simulink model "ModeAdjust"  (R2018b)
settings: Solver=FixedStepDiscrete  StartTime=0.0  StopTime=inf  FixedStep=0.01  RelTol=1e-3
undefined symbols (not defined in the file or in its folder): IfKeSMSbSeatMovBkRclnEnable_Val, IfKeSMSbSeatMovFrwdBkwdEnable_Val, IfKeSMSbSeatMovFtrstEnable_Val, IfKeSMSbSeatMovHdrstFrwdBkwdEnable_Val, IfKeSMSbSeatMovHdUpwdDnwdEnable_Val, IfKeSMSbSeatMovLgrstEnable_Val, IfKeSMSbSeatMovLtwdRtwdEnable_Val, IfVeSMSeStNumConfig, KeSMSbArmscreenMovEnable_Val, KeSMSbSeatMovLgrstExpdEnable_Val, KeSMSuFirstRwStBackPosDelta_Val, KeSMSuFirstRwStBackPosTolr_Val, KeSMSuFirstRwStCushFrntPosDelta_Val, KeSMSuFirstRwStCushFrntPosTolr_Val, KeSMSuFirstRwStCushRePosDelta_Val, KeSMSuFirstRwStCushRePosTolr_Val, KeSMSuFirstRwStFootrestPosDelta_Val, KeSMSuFirstRwStFootrestPosTolr_Val, KeSMSuFirstRwStFwdBkwdPosDelta_Val, KeSMSuFirstRwStFwdBkwdPosTolr_Val, KeSMSuMdMotFinshdTm_Val, KeSMSuMdRetryTm1_Val, KeSMSuModeReqDurgTm_Val, KeSMSuSecRwStArmTochPosDelta_Val, KeSMSuSecRwStArmTochPosTolr_Val, KeSMSuSecRwStBackPosDelta_Val, KeSMSuSecRwStBackPosTolr_Val, KeSMSuSecRwStFtrstUpwdDnwdPosDelta_Val, KeSMSuSecRwStFtrstUpwdDnwdPosTolr_Val, KeSMSuSecRwStFwdBkwdPosDelta_Val, KeSMSuSecRwStFwdBkwdPosTolr_Val, KeSMSuSecRwStHeadrestFwdBkwdPosDelta_Val, KeSMSuSecRwStHeadrestFwdBkwdPosTolr_Val, KeSMSuSecRwStHeadrestUpwdDwnwdPosDelta_Val, KeSMSuSecRwStHeadrestUpwdDwnwdPosTolr_Val, KeSMSuSecRwStLegrestInOutPosDelta_Val, KeSMSuSecRwStLegrestInOutPosTolr_Val, KeSMSuSecRwStLegrestUpwdDwnwdPosDelta_Val, KeSMSuSecRwStLegrestUpwdDwnwdPosTolr_Val, KeSMSuSecRwStLwdRwdPosDelta_Val, KeSMSuSecRwStLwdRwdPosTolr_Val, KeSMSuSecRwStVIPFtrstRefAngle_Val, KeSMSuThirdRwStFwdBkwdPosDelta_Val, KeSMSuThirdRwStFwdBkwdPosTolr_Val, KeSMSuThrdRwCushFoldPosDelta_Val, KeSMSuThrdRwCushFoldPosTolr_Val, KeSMSuThrdRwStBackPosDelta_Val, KeSMSuThrdRwStBackPosTolr_Val, KeSMSw4SLegrstCloseMdSecRwLtStFtrstUpwdDnwdPos_Val, KeSMSw4SLegrstCloseMdSecRwLtStFtrstUpwdDnwdPosMax_Val, KeSMSw4SLegrstCloseMdSecRwLtStFtrstUpwdDnwdPosMin_Val, KeSMSw4SLegrstCloseMdSecRwLtStLgrstOtwdInwdPos_Val, KeSMSw4SLegrstCloseMdSecRwLtStLgrstOtwdInwdPosMax_Val, KeSMSw4SLegrstCloseMdSecRwLtStLgrstOtwdInwdPosMin_Val, KeSMSw4SLegrstCloseMdSecRwLtStLgrstUpwdDnwdPos_Val, KeSMSw4SLegrstCloseMdSecRwLtStLgrstUpwdDnwdPosMax_Val, KeSMSw4SLegrstCloseMdSecRwLtStLgrstUpwdDnwdPosMin_Val, KeSMSw4SLegrstCloseMdSecRwRtStFtrstUpwdDnwdPos_Val, KeSMSw4SLegrstCloseMdSecRwRtStFtrstUpwdDnwdPosMax_Val, KeSMSw4SLegrstCloseMdSecRwRtStFtrstUpwdDnwdPosMin_Val ... (+1138)
libraries: Lib x401
(part 20 of 35)

== system ModeAdjust/ModeAdjustRunnable_sys/ModeAdjust/RecoveryL/R2Lt ==
  note: 2L 扶手屏位置
  note: %1锁，2未锁
  Mode_Trig : Inport
  Step1En : Inport  Port=2
  SecRwLtStsPoss : Inport  Port=3
  SecRwLtStPossV : Inport  Port=4
  SecRwRtStChldLkRsp_L : Inport  Port=5
  ModeStCalib_2L : Inport  Port=6
  StConfig : Inport  Port=7
  Bus Creator : BusCreator  Inputs=9  OutDataTypeStr=Bus: SecRwLfSeatPos
  Bus Selector : BusSelector  OutputSignals=IfVeSMSuSecRwLtStBkReclnUpwdDnwdPos_Val_read,IfVeSMSuSecRwLtStFrwdBkwdPos_Val_read,IfVeSMSuSecRwLtStHPassStUpwdDnwdPos_Val_read,IfVeSMSuSecRwLtStLgrstUpwdDnwdPos_Val_read,IfVeSMSuSecRwLtStLtwdRtwdPos_Val_read,IfVeSMSuSecRwLtStArmScrnPos_Val_read
  Bus Selector1 : BusSelector  OutputSignals=IfVeSMSuSecRwLtStBkReclnUpwdDnwdPosV_Val_read,IfVeSMSuSecRwLtStFrwdBkwdPosV_Val_read,IfVeSMSuSecRwLtStHPassStUpwdDnwdPosV_Val_read,IfVeSMSuSecRwLtStLgrstUpwdDnwdPosV_Val_read,IfVeSMSuSecRwLtStLtwdRtwdPosV_Val_read,IfVeSMSuSecRwLtStArmScrnPosV_Val_read
  Bus Selector2 : BusSelector  OutputSignals=ArmScrnPos,ArmScrnPosMax,ArmScrnPosMin,BkReclnUpwdDnwdPos,BkReclnUpwdDnwdPosMax,BkReclnUpwdDnwdPosMin,FrwdBkwdPos,FrwdBkwdPosMax,FrwdBkwdPosMin,HdrstUpwdPos,HdrstUpwdPosMax,HdrstUpwdPosMin,LgrstUpwdPos,LgrstUpwdPosMax,LgrstUpwdPosMin,LtwdRtwdPos,LtwdRtwdPosMax,LtwdRtwdPosMin
  Bus Selector3 : BusSelector  OutputSignals=RecoveryMdSecRwLtSt
  Bus Selector4 : BusSelector  OutputSignals=BkReclnUpwdDnwdMovConfig,ArmTouchMovConfig,FrwdBkwdMovConfig,LgrstUpwdMovConfig,LtwdRtwdMovConfig
  Delay2 : Delay  DelayLength=1
  Delay3 : Delay  DelayLength=1
  Logical Operator1 : Logic  AllPortsSameDT=off  OutDataTypeStr=boolean
  Logical Operator2 : Logic  AllPortsSameDT=off  OutDataTypeStr=boolean
  Logical Operator3 : Logic  Operator=OR  AllPortsSameDT=off  OutDataTypeStr=boolean
  PA_KeSMSuMdMotFinshdTm_Val : Constant  Value=KeSMSuMdMotFinshdTm_Val
  PA_KeSMSuMdRetryTm1_Val : Constant  Value=KeSMSuMdRetryTm1_Val
  PA_KeSMSuModeReqDurgTm_Val : Constant  Value=KeSMSuModeReqDurgTm_Val
  PA_KeSMSuSecRwStArmTochPosDelta_Val : Constant  Value=KeSMSuSecRwStArmTochPosDelta_Val
  PA_KeSMSuSecRwStBackPosDelta_Val : Constant  Value=KeSMSuSecRwStBackPosDelta_Val
  PA_KeSMSuSecRwStFwdBkwdPosDelta_Val : Constant  Value=KeSMSuSecRwStFwdBkwdPosDelta_Val
  PA_KeSMSuSecRwStLegrestUpwdDwnwdPosDelta_Val : Constant  Value=KeSMSuSecRwStLegrestUpwdDwnwdPosDelta_Val
  PA_KeSMSuSecRwStLwdRwdPosDelta_Val : Constant  Value=KeSMSuSecRwStLwdRwdPosDelta_Val
  PA_KeSMSwDltTrgtPos_Val{1,3,7..8,12,18..21} (9 alike) : Constant  Value=KeSMSwPosInvalidVal_Val
  PA_KeSMSwDltTrgtPos_Val2 : Constant  Value=SeatChldLkSt.ChldLkSt_Unlock
  PA_KeSMSwDltTrgtPos_Val4 : Constant  OutDataTypeStr=boolean
  PA_KeSMSwDltTrgtPos_Val5 : Constant  Value=0  OutDataTypeStr=boolean
  PA_KeSMSwDltTrgtPos_Val9 : Constant  Value=0  OutDataTypeStr=boolean
  Relational Operator : RelationalOperator  Operator=~=  OutDataTypeStr=boolean  RndMeth=Simplest
  SecRwLtStBkReclnUpwdDnwd_Lt_Step1 : Lib/CommonUsed  SystemSampleTime=-1
  SecRwLtStLgrstUpwd_Lt_Step3 : Lib/CommonUsed  SystemSampleTime=-1
  R2Lt_Recovery_Ini : Outport
  R2Lt_Recovery_done : Outport  Port=2
  R2Lt_TrgtPoss : Outport  Port=3  VectorParamsAs1DForOutWhenUnconnected=on
  IfVeSMSuSecRwLtStRclCmdSrv_Val_writeRaw : Outport  Port=4
  wires:
  PA_KeSMSwDltTrgtPos_Val4/1 -> IfVeSMSuSecRwLtStRclCmdSrv_Val_writeRaw/1
  Delay3/1 -> [Step1done_1]
  SecRwLtStLgrstUpwd_Lt_Step3/1 -> [Step3_2_ini]
  Logical Operator2/1 -> Logical Operator3/1, R2Lt_Recovery_Ini/1
  [K_BkReclnUpwdDnwdPosMax] -> SecRwLtStBkReclnUpwdDnwd_Lt_Step1/5
  [Trig] -> SecRwLtStBkReclnUpwdDnwd_Lt_Step1/1
  Mode_Trig/1 -> [Trig]
  [KeSMSuSecRwStBackPosDelta_Val] -> SecRwLtStBkReclnUpwdDnwd_Lt_Step1/7
  [K_BkReclnUpwdDnwdPosMin] -> SecRwLtStBkReclnUpwdDnwd_Lt_Step1/4
  SecRwLtStBkReclnUpwdDnwd_Lt_Step1/2 -> [Step1_1_ArrivedTarPos]
  [SecRwLtStBkReclnUpwdDnwdPos] -> SecRwLtStBkReclnUpwdDnwd_Lt_Step1/3
  [K_BkReclnUpwdDnwdPos] -> SecRwLtStBkReclnUpwdDnwd_Lt_Step1/6
  PA_KeSMSwDltTrgtPos_Val3/1 -> SecRwLtStBkReclnUpwdDnwd_Lt_Step1/10
  SecRwLtStBkReclnUpwdDnwd_Lt_Step1/3 -> [R2Lt_BkReclnUpwdDnwd_TarPos]
  [ChildLocker] -> SecRwLtStBkReclnUpwdDnwd_Lt_Step1/9
  [Tick] -> SecRwLtStBkReclnUpwdDnwd_Lt_Step1/11
  Bus Selector1/3 -> [SecRwLtStHPassStUpwdDnwdPosV]  "<IfVeSMSuSecRwLtStHPassStUpwdDnwdPosV_Val_read>"
  Bus Selector/5 -> [SecRwLtStLtwdRtwdPos]  "<IfVeSMSuSecRwLtStLtwdRtwdPos_Val_read>"
  SecRwLtStsPoss/1 -> Bus Selector/1
  Bus Selector1/4 -> [SecRwLtStLgrstUpwdDnwdPosV]  "<IfVeSMSuSecRwLtStLgrstUpwdDnwdPosV_Val_read>"
  SecRwLtStPossV/1 -> Bus Selector1/1
  Bus Selector/3 -> [SecRwLtStHPassStUpwdDnwdPos]  "<IfVeSMSuSecRwLtStHPassStUpwdDnwdPos_Val_read>"
  Bus Selector1/5 -> [SecRwLtStLtwdRtwdPosV]  "<IfVeSMSuSecRwLtStLtwdRtwdPosV_Val_read>"
  Bus Selector/4 -> [SecRwLtStLgrstUpwdDnwdPos]  "<IfVeSMSuSecRwLtStLgrstUpwdDnwdPos_Val_read>"
  Bus Selector/2 -> [SecRwLtStFrwdBkwdPos]  "<IfVeSMSuSecRwLtStFrwdBkwdPos_Val_read>"
  Bus Selector1/1 -> [SecRwLtStBkReclnUpwdDnwdPosV]  "<IfVeSMSuSecRwLtStBkReclnUpwdDnwdPosV_Val_read>"
  Bus Selector1/2 -> [SecRwLtStFrwdBkwdPosV]  "<IfVeSMSuSecRwLtStFrwdBkwdPosV_Val_read>"
  Bus Selector/1 -> [SecRwLtStBkReclnUpwdDnwdPos]  "<IfVeSMSuSecRwLtStBkReclnUpwdDnwdPos_Val_read>"
  SecRwRtStChldLkRsp_L/1 -> Relational Operator/1
  PA_KeSMSwDltTrgtPos_Val2/1 -> Relational Operator/2
  Relational Operator/1 -> [ChildLocker]
  [Trig] -> SecRwLtStLgrstUpwd_Lt_Step3/1
  [StepEn] -> SecRwLtStLgrstUpwd_Lt_Step3/2
  [K_LgrstUpwdPosMin] -> SecRwLtStLgrstUpwd_Lt_Step3/4
  [K_LgrstUpwdPosMax] -> SecRwLtStLgrstUpwd_Lt_Step3/5
  [K_LgrstUpwdPos] -> SecRwLtStLgrstUpwd_Lt_Step3/6
  [SecRwLtStLgrstUpwdDnwdPos] -> SecRwLtStLgrstUpwd_Lt_Step3/3
  [SecRwLtStBkReclnUpwdDnwdPosV] -> SecRwLtStBkReclnUpwdDnwd_Lt_Step1/8
  [KeSMSuSecRwStLegrestUpwdDwnwdPosDelta_Val] -> SecRwLtStLgrstUpwd_Lt_Step3/7
  [SecRwLtStLgrstUpwdDnwdPosV] -> SecRwLtStLgrstUpwd_Lt_Step3/8
  [ChildLocker] -> SecRwLtStLgrstUpwd_Lt_Step3/9
  PA_KeSMSwDltTrgtPos_Val12/1 -> SecRwLtStLgrstUpwd_Lt_Step3/10
  [Tick] -> SecRwLtStLgrstUpwd_Lt_Step3/11
  SecRwLtStLgrstUpwd_Lt_Step3/2 -> [Step1_2_ArrivedTarPos]
  SecRwLtStLgrstUpwd_Lt_Step3/3 -> [R2Lt_LgrstUpwd_TarPos]
  SecRwLtStLgrstUpwd_Lt_Step3/4 -> [Step3done]
  SecRwLtStBkReclnUpwdDnwd_Lt_Step1/1 -> [Step3_1_ini]
  SecRwLtStBkReclnUpwdDnwd_Lt_Step1/4 -> Delay3/1
  PA_KeSMSwDltTrgtPos_Val21/1 -> Bus Creator/6  "SecRwLtStHdrstUpwdDnwdTrgtPos"
  Bus Creator/1 -> R2Lt_TrgtPoss/1
  [R2Lt_LgrstUpwd_TarPos] -> Bus Creator/7  "SecRwLtStLgrstUpwdDnwdTrgtPos"
  PA_KeSMSwDltTrgtPos_Val19/1 -> Bus Creator/3  "SecRwLtStCshnFrntUpwdDnwdTrgtPos"
  PA_KeSMSwDltTrgtPos_Val1/1 -> Bus Creator/8  "SecRwLtStLtwdRtwdTrgtPos"
  PA_KeSMSwDltTrgtPos_Val18/1 -> Bus Creator/2  "SecRwLtStBlstOtwdInwdTrgtPos"
  [R2Lt_BkReclnUpwdDnwd_TarPos] -> Bus Creator/1  "SecRwLtStBkReclnUpwdDnwdTrgtPos"
  PA_KeSMSwDltTrgtPos_Val8/1 -> Bus Creator/5  "SecRwLtStFrwdBkwdTrgtPos"
  PA_KeSMSwDltTrgtPos_Val20/1 -> Bus Creator/4  "SecRwLtStCshnRrUpwdDnwdTrgtPos"
  Step1En/1 -> [StepEn]
  [Step3_1_ini] -> Logical Operator2/1
  [Step3_2_ini] -> Logical Operator2/2
  [Step1done_1] -> Logical Operator1/1
  [Step3done] -> Logical Operator1/2
  Logical Operator3/1 -> R2Lt_Recovery_done/1
  [StepEn] -> SecRwLtStBkReclnUpwdDnwd_Lt_Step1/2
  Logical Operator1/1 -> Delay2/1
  Delay2/1 -> Logical Operator3/2
  PA_KeSMSuModeReqDurgTm_Val/1 -> [Tick]
  PA_KeSMSwDltTrgtPos_Val7/1 -> Bus Creator/9  "SecRwLtStArmScrnTrgtPos"
  PA_KeSMSuSecRwStFwdBkwdPosDelta_Val/1 -> [KeSMSuSecRwStFwdBkwdPosDelta_Val]
  PA_KeSMSuSecRwStLwdRwdPosDelta_Val/1 -> [KeSMSuSecRwStLwdRwdPosDelta_Val]
  PA_KeSMSuSecRwStArmTochPosDelta_Val/1 -> [KeSMSuSecRwStArmTochPosDelta_Val]
  PA_KeSMSuSecRwStBackPosDelta_Val/1 -> [KeSMSuSecRwStBackPosDelta_Val]
  PA_KeSMSuSecRwStLegrestUpwdDwnwdPosDelta_Val/1 -> [KeSMSuSecRwStLegrestUpwdDwnwdPosDelta_Val]
  PA_KeSMSuMdMotFinshdTm_Val/1 -> [KeSMSuMdMotFinshdTm_Val]
  [KeSMSuMdMotFinshdTm_Val] -> SecRwLtStBkReclnUpwdDnwd_Lt_Step1/12
  [KeSMSuMdMotFinshdTm_Val] -> SecRwLtStLgrstUpwd_Lt_Step3/12
  Bus Selector/6 -> [R2LtStArmScrnPos]  "<IfVeSMSuSecRwLtStArmScrnPos_Val_read>"
  Bus Selector1/6 -> [R2LtStArmScrnPosV]  "<IfVeSMSuSecRwLtStArmScrnPosV_Val_read>"
  Bus Selector2/1 -> [K_ArmScrnPos]  "<ArmScrnPos>"
  Bus Selector2/18 -> [K_LtwdRtwdPosMin]  "<LtwdRtwdPosMin>"
  Bus Selector2/16 -> [K_LtwdRtwdPos]  "<LtwdRtwdPos>"
  Bus Selector2/15 -> [K_LgrstUpwdPosMin]  "<LgrstUpwdPosMin>"
  Bus Selector2/17 -> [K_LtwdRtwdPosMax]  "<LtwdRtwdPosMax>"
  Bus Selector2/12 -> [K_HdrstUpwdPosMin]  "<HdrstUpwdPosMin>"
  Bus Selector2/13 -> [K_LgrstUpwdPos]  "<LgrstUpwdPos>"
  Bus Selector2/11 -> [K_HdrstUpwdPosMax]  "<HdrstUpwdPosMax>"
  Bus Selector2/14 -> [K_LgrstUpwdPosMax]  "<LgrstUpwdPosMax>"
  Bus Selector2/10 -> [K_HdrstUpwdPos]  "<HdrstUpwdPos>"
  Bus Selector2/4 -> [K_BkReclnUpwdDnwdPos]  "<BkReclnUpwdDnwdPos>"
  Bus Selector2/9 -> [K_FrwdBkwdPosMin]  "<FrwdBkwdPosMin>"
  Bus Selector2/5 -> [K_BkReclnUpwdDnwdPosMax]  "<BkReclnUpwdDnwdPosMax>"
  Bus Selector2/8 -> [K_FrwdBkwdPosMax]  "<FrwdBkwdPosMax>"
  Bus Selector3/1 -> Bus Selector2/1  "<RecoveryMdSecRwLtSt>"
  Bus Selector2/7 -> [K_FrwdBkwdPos]  "<FrwdBkwdPos>"
  Bus Selector2/3 -> [K_ArmScrnPosMin]  "<ArmScrnPosMin>"
  Bus Selector2/2 -> [K_ArmScrnPosMax]  "<ArmScrnPosMax>"
  Bus Selector2/6 -> [K_BkReclnUpwdDnwdPosMin]  "<BkReclnUpwdDnwdPosMin>"
  ModeStCalib_2L/1 -> Bus Selector3/1
  StConfig/1 -> Bus Selector4/1
  Bus Selector4/3 -> [FrwdBkwdMovConfig]  "<FrwdBkwdMovConfig>"
  Bus Selector4/5 -> [LtwdRtwdMovConfig]  "<LtwdRtwdMovConfig>"
  Bus Selector4/4 -> [LgrstUpwdMovConfig]  "<LgrstUpwdMovConfig>"
  Bus Selector4/2 -> [ArmTouchMovConfig]  "<ArmTouchMovConfig>"
  Bus Selector4/1 -> [BkReclnUpwdDnwdMovConfig]  "<BkReclnUpwdDnwdMovConfig>"
  PA_KeSMSwDltTrgtPos_Val9/1 -> SecRwLtStLgrstUpwd_Lt_Step3/13
  [LgrstUpwdMovConfig] -> SecRwLtStLgrstUpwd_Lt_Step3/14
  [CntLow] -> SecRwLtStLgrstUpwd_Lt_Step3/15
  PA_KeSMSuMdRetryTm1_Val/1 -> [CntLow]
  [BkReclnUpwdDnwdMovConfig] -> SecRwLtStBkReclnUpwdDnwd_Lt_Step1/14
  PA_KeSMSwDltTrgtPos_Val5/1 -> SecRwLtStBkReclnUpwdDnwd_Lt_Step1/13
  [CntLow] -> SecRwLtStBkReclnUpwdDnwd_Lt_Step1/15

== system ModeAdjust/ModeAdjustRunnable_sys/ModeAdjust/RecoveryR/Pass ==
  note: %1锁，2未锁
  Mode_Trig : Inport
  Step1En : Inport  Port=2
  PassStPoss : Inport  Port=3
  PassStPossV : Inport  Port=4
  ModeStCalib_Pass : Inport  Port=5
  StConfig : Inport  Port=6
  SecRwRtStChldLkRsp_L : Inport  Port=7
  Bus Creator : BusCreator  Inputs=8  OutDataTypeStr=Bus: PasSeatPos
  Bus Selector : BusSelector  OutputSignals=IfVeSMSuPassStBkReclnUpwdDnwdPos_Val_read,IfVeSMSuPassStCshnFrntUpwdDnwdPos_Val_read,IfVeSMSuPassStCshnRrUpwdDnwdPos_Val_read,IfVeSMSuPassStFrwdBkwdPos_Val_read,IfVeSMSuPassStFtUpwdDnwdPos_Val_read
  Bus Selector1 : BusSelector  OutputSignals=IfVeSMSuPassStBkReclnUpwdDnwdPosV_Val_read,IfVeSMSuPassStCshnFrntUpwdDnwdPosV_Val_read,IfVeSMSuPassStCshnRrUpwdDnwdPosV_Val_read,IfVeSMSuPassStFrwdBkwdPosV_Val_read,IfVeSMSuPassStFtUpwdDnwdPosV_Val_read
  Bus Selector2 : BusSelector  OutputSignals=BkReclnUpwdDnwdPos,BkReclnUpwdDnwdPosMax,BkReclnUpwdDnwdPosMin,FrwdBkwdPos,FrwdBkwdPosMax,FrwdBkwdPosMin,FtUpwdDnwdPos,FtUpwdDnwdPosMax,FtUpwdDnwdPosMin
  Bus Selector3 : BusSelector  OutputSignals=RecvPassSt
  Bus Selector4 : BusSelector  OutputSignals=BkReclnUpwdDnwdMovConfig,FrwdBkwdMovConfig,FtUpwdDnwdMovConfig
  Logical Operator : Logic  Operator=OR  AllPortsSameDT=off  OutDataTypeStr=boolean
  PA_KeSMSuFirstRwStBackPosDelta_Val : Constant  Value=KeSMSuFirstRwStBackPosDelta_Val
  PA_KeSMSuFirstRwStFootrestPosDelta_Val : Constant  Value=KeSMSuFirstRwStFootrestPosDelta_Val
  PA_KeSMSuFirstRwStFwdBkwdPosDelta_Val : Constant  Value=KeSMSuFirstRwStFwdBkwdPosDelta_Val
  PA_KeSMSuMdMotFinshdTm_Val : Constant  Value=KeSMSuMdMotFinshdTm_Val
  PA_KeSMSuMdRetryTm1_Val : Constant  Value=KeSMSuMdRetryTm1_Val
  PA_KeSMSuModeReqDurgTm_Val : Constant  Value=KeSMSuModeReqDurgTm_Val
  PA_KeSMSwDltTrgtPos_Val{1..2,12,14..18} (8 alike) : Constant  Value=KeSMSwPosInvalidVal_Val
  PA_KeSMSwDltTrgtPos_Val3 : Constant  Value=SeatChldLkSt.ChldLkSt_Unlock
  PA_KeSMSwDltTrgtPos_Val4 : Constant  Value=0  OutDataTypeStr=boolean
  PA_KeSMSwDltTrgtPos_Val7 : Constant  OutDataTypeStr=boolean
  PassStFtUpwdDnwd_Step1 : Lib/CommonUsed  SystemSampleTime=-1
  Relational Operator : RelationalOperator  Operator=~=  OutDataTypeStr=boolean  RndMeth=Simplest
  Unit Delay : UnitDelay  SampleTime=-1
  Pass_Step1_ini : Outport
  Pass_Step1_done : Outport  Port=2
  PassStTrgtPoss : Outport  Port=3  VectorParamsAs1DForOutWhenUnconnected=on
  IfVeSMSuPassStRclCmdSrv_Val_writeRaw : Outport  Port=4
  wires:
  [PassStFtUpwdDnwd_TarPos] -> Bus Creator/6  "PassStFtUpwdDnwdTrgtPos"
  PA_KeSMSwDltTrgtPos_Val15/1 -> Bus Creator/3  "PassStCshnFrntUpwdDnwdTrgtPos"
  PA_KeSMSwDltTrgtPos_Val14/1 -> Bus Creator/2  "PassStBlstOtwdInwdTrgtPos"
  PA_KeSMSwDltTrgtPos_Val2/1 -> Bus Creator/1  "PassStBkReclnUpwdDnwdTrgtPos"
  PA_KeSMSwDltTrgtPos_Val18/1 -> Bus Creator/8  "PassStLgrstUpwdDnwdTrgtPos"
  PA_KeSMSwDltTrgtPos_Val17/1 -> Bus Creator/7  "PassStHdrstUpwdDnwdTrgtPos"
  PA_KeSMSwDltTrgtPos_Val1/1 -> Bus Creator/5  "PassStFrwdBkwdTrgtPos"
  PA_KeSMSwDltTrgtPos_Val16/1 -> Bus Creator/4  "PassStCshnRrUpwdDnwdTrgtPos"
  Bus Creator/1 -> PassStTrgtPoss/1
  [FtUpwdDnwd_Step1_ini] -> Pass_Step1_ini/1
  PassStFtUpwdDnwd_Step1/1 -> [FtUpwdDnwd_Step1_ini]
  Bus Selector1/5 -> [PassStFtUpwdDnwdPosV]  "<IfVeSMSuPassStFtUpwdDnwdPosV_Val_read>"
  PassStPoss/1 -> Bus Selector/1
  Bus Selector1/1 -> [PassStBkReclnUpwdDnwdPosV]  "<IfVeSMSuPassStBkReclnUpwdDnwdPosV_Val_read>"
  Bus Selector1/4 -> [PassStFrwdBkwdPosV]  "<IfVeSMSuPassStFrwdBkwdPosV_Val_read>"
  Bus Selector/4 -> [PassStFrwdBkwdPos]  "<IfVeSMSuPassStFrwdBkwdPos_Val_read>"
  Bus Selector/1 -> [PassStBkReclnUpwdDnwdPos]  "<IfVeSMSuPassStBkReclnUpwdDnwdPos_Val_read>"
  Bus Selector1/2 -> [PassStCshnFrntUpwdDnwdPosV]  "<IfVeSMSuPassStCshnFrntUpwdDnwdPosV_Val_read>"
  Bus Selector/3 -> [PassStCshnRrUpwdDnwdPos]  "<IfVeSMSuPassStCshnRrUpwdDnwdPos_Val_read>"
  PassStPossV/1 -> Bus Selector1/1
  Bus Selector1/3 -> [PassStCshnRrUpwdDnwdPosV]  "<IfVeSMSuPassStCshnRrUpwdDnwdPosV_Val_read>"
  Bus Selector/5 -> [PassStFtUpwdDnwdPos]  "<IfVeSMSuPassStFtUpwdDnwdPos_Val_read>"
  Bus Selector/2 -> [PassStCshnFrntUpwdDnwdPos]  "<IfVeSMSuPassStCshnFrntUpwdDnwdPos_Val_read>"
  PassStFtUpwdDnwd_Step1/4 -> [Step1done_2]
  PassStFtUpwdDnwd_Step1/3 -> [PassStFtUpwdDnwd_TarPos]
  PassStFtUpwdDnwd_Step1/2 -> [Step1_2_ArrivedTarPos]
  [Tick] -> PassStFtUpwdDnwd_Step1/11
  PA_KeSMSwDltTrgtPos_Val12/1 -> PassStFtUpwdDnwd_Step1/10
  [ChildLocker] -> PassStFtUpwdDnwd_Step1/9
  [PassStFtUpwdDnwdPosV] -> PassStFtUpwdDnwd_Step1/8
  [KeSMSuFirstRwStFootrestPosDelta_Val] -> PassStFtUpwdDnwd_Step1/7
  [PassStFtUpwdDnwdPos] -> PassStFtUpwdDnwd_Step1/3
  [K_FtUpwdDnwdPos] -> PassStFtUpwdDnwd_Step1/6
  [K_FtUpwdDnwdPosMax] -> PassStFtUpwdDnwd_Step1/5
  [K_FtUpwdDnwdPosMin] -> PassStFtUpwdDnwd_Step1/4
  [Step1En] -> PassStFtUpwdDnwd_Step1/2
  [Trig] -> PassStFtUpwdDnwd_Step1/1
  Mode_Trig/1 -> [Trig]
  Step1En/1 -> [Step1En]
  PA_KeSMSwDltTrgtPos_Val7/1 -> IfVeSMSuPassStRclCmdSrv_Val_writeRaw/1
  PA_KeSMSuModeReqDurgTm_Val/1 -> [Tick]
  PA_KeSMSuFirstRwStBackPosDelta_Val/1 -> [KeSMSuFirstRwStBackPosDelta_Val]
  PA_KeSMSuFirstRwStFwdBkwdPosDelta_Val/1 -> [KeSMSuFirstRwStFwdBkwdPosDelta_Val]
  PA_KeSMSuMdMotFinshdTm_Val/1 -> [KeSMSuMdMotFinshdTm_Val]
  PA_KeSMSuFirstRwStFootrestPosDelta_Val/1 -> [KeSMSuFirstRwStFootrestPosDelta_Val]
  [KeSMSuMdMotFinshdTm_Val] -> PassStFtUpwdDnwd_Step1/12
  Bus Selector2/2 -> [K_BkReclnUpwdDnwdPosMax]  "<BkReclnUpwdDnwdPosMax>"
  Bus Selector2/9 -> [K_FtUpwdDnwdPosMin]  "<FtUpwdDnwdPosMin>"
  Bus Selector3/1 -> Bus Selector2/1  "<RecvPassSt>"
  ModeStCalib_Pass/1 -> Bus Selector3/1
  Bus Selector2/6 -> [K_FrwdBkwdPosMin]  "<FrwdBkwdPosMin>"
  Bus Selector2/3 -> [K_BkReclnUpwdDnwdPosMin]  "<BkReclnUpwdDnwdPosMin>"
  Bus Selector2/4 -> [K_FrwdBkwdPos]  "<FrwdBkwdPos>"
  Bus Selector2/7 -> [K_FtUpwdDnwdPos]  "<FtUpwdDnwdPos>"
  Bus Selector2/5 -> [K_FrwdBkwdPosMax]  "<FrwdBkwdPosMax>"
  Bus Selector2/1 -> [K_BkReclnUpwdDnwdPos]  "<BkReclnUpwdDnwdPos>"
  Bus Selector2/8 -> [K_FtUpwdDnwdPosMax]  "<FtUpwdDnwdPosMax>"
  PA_KeSMSwDltTrgtPos_Val4/1 -> PassStFtUpwdDnwd_Step1/13
  Bus Selector4/1 -> [BkReclnUpwdDnwdMovConfig]  "<BkReclnUpwdDnwdMovConfig>"
  Bus Selector4/3 -> [FtUpwdDnwdMovConfig]  "<FtUpwdDnwdMovConfig>"
  Bus Selector4/2 -> [FrwdBkwdMovConfig]  "<FrwdBkwdMovConfig>"
  StConfig/1 -> Bus Selector4/1
  [FtUpwdDnwdMovConfig] -> PassStFtUpwdDnwd_Step1/14
  [FtUpwdDnwd_Step1_ini] -> Logical Operator/1
  Logical Operator/1 -> Pass_Step1_done/1
  Unit Delay/1 -> Logical Operator/2
  [Step1done_2] -> Unit Delay/1
  Relational Operator/1 -> [ChildLocker]
  SecRwRtStChldLkRsp_L/1 -> Relational Operator/1
  PA_KeSMSwDltTrgtPos_Val3/1 -> Relational Operator/2
  [CntLow] -> PassStFtUpwdDnwd_Step1/15
  PA_KeSMSuMdRetryTm1_Val/1 -> [CntLow]

== system ModeAdjust/ModeAdjustRunnable_sys/ModeAdjust/RecoveryR/R2Rt ==
  note: %1锁，2未锁
  Mode_Trig : Inport
  Step1En : Inport  Port=2
  SecRwRtStPoss : Inport  Port=3
  SecRwRtStPossV : Inport  Port=4
  SecRwRtStChldLkRsp_L : Inport  Port=5
  ModeStCalib_2R : Inport  Port=6
  StConfig : Inport  Port=7
  Bus Creator : BusCreator  Inputs=9  OutDataTypeStr=Bus: SecRwRtSeatPos
  Bus Selector : BusSelector  OutputSignals=IfVeSMSuSecRwRtStBkReclnUpwdDnwdPos_Val_read,IfVeSMSuSecRwRtStFrwdBkwdPos_Val_read,IfVeSMSuSecRwRtStHPassStUpwdDnwdPos_Val_read,IfVeSMSuSecRwRtStLgrstUpwdDnwdPos_Val_read,IfVeSMSuSecRwRtStLtwdRtwdPos_Val_read,SecRwRtStArmScrnPos_Val_read
  Bus Selector1 : BusSelector  OutputSignals=IfVeSMSuSecRwRtStBkReclnUpwdDnwdPosV_Val_read,IfVeSMSuSecRwRtStFrwdBkwdPosV_Val_read,IfVeSMSuSecRwRtStHPassStUpwdDnwdPosV_Val_read,IfVeSMSuSecRwRtStLgrstUpwdDnwdPosV_Val_read,IfVeSMSuSecRwRtStLtwdRtwdPosV_Val_read,SecRwRtStArmScrnPosV_Val_read
  Bus Selector2 : BusSelector  OutputSignals=ArmScrnPos,ArmScrnPosMax,ArmScrnPosMin,BkReclnUpwdDnwdPos,BkReclnUpwdDnwdPosMax,BkReclnUpwdDnwdPosMin,FrwdBkwdPos,FrwdBkwdPosMax,FrwdBkwdPosMin,HdrstUpwdPos,HdrstUpwdPosMax,HdrstUpwdPosMin,LgrstUpwdPos,LgrstUpwdPosMax,LgrstUpwdPosMin,LtwdRtwdPos,LtwdRtwdPosMax,LtwdRtwdPosMin
  Bus Selector3 : BusSelector  OutputSignals=RecoveryMdSecRwRtSt
  Bus Selector4 : BusSelector  OutputSignals=BkReclnUpwdDnwdMovConfig,ArmTouchMovConfig,FrwdBkwdMovConfig,LgrstUpwdMovConfig,LtwdRtwdMovConfig
  Logical Operator1 : Logic  AllPortsSameDT=off  OutDataTypeStr=boolean
  Logical Operator2 : Logic  Operator=OR  AllPortsSameDT=off  OutDataTypeStr=boolean
  Logical Operator6 : Logic  AllPortsSameDT=off  OutDataTypeStr=boolean
  PA_KeSMSuMdMotFinshdTm_Val : Constant  Value=KeSMSuMdMotFinshdTm_Val
  PA_KeSMSuMdRetryTm1_Val : Constant  Value=KeSMSuMdRetryTm1_Val
  PA_KeSMSuModeReqDurgTm_Val : Constant  Value=KeSMSuModeReqDurgTm_Val
  PA_KeSMSuSecRwStArmTochPosDelta_Val : Constant  Value=KeSMSuSecRwStArmTochPosDelta_Val
  PA_KeSMSuSecRwStBackPosDelta_Val : Constant  Value=KeSMSuSecRwStBackPosDelta_Val
  PA_KeSMSuSecRwStFwdBkwdPosDelta_Val : Constant  Value=KeSMSuSecRwStFwdBkwdPosDelta_Val
  PA_KeSMSuSecRwStLegrestUpwdDwnwdPosDelta_Val : Constant  Value=KeSMSuSecRwStLegrestUpwdDwnwdPosDelta_Val
  PA_KeSMSuSecRwStLwdRwdPosDelta_Val : Constant  Value=KeSMSuSecRwStLwdRwdPosDelta_Val
  PA_KeSMSwDltTrgtPos_Val{1,3..5,12,19..22} (9 alike) : Constant  Value=KeSMSwPosInvalidVal_Val
  PA_KeSMSwDltTrgtPos_Val18 : Constant  OutDataTypeStr=boolean
  PA_KeSMSwDltTrgtPos_Val2 : Constant  Value=SeatChldLkSt.ChldLkSt_Unlock
  PA_KeSMSwDltTrgtPos_Val6 : Constant  Value=0  OutDataTypeStr=boolean
  PA_KeSMSwDltTrgtPos_Val8 : Constant  Value=0  OutDataTypeStr=boolean
  R2RtSt_BkReclnUpwdDnwd_Step1 : Lib/CommonUsed  SystemSampleTime=-1
  R2RtSt_LgrstUpwd_Step3 : Lib/CommonUsed  SystemSampleTime=-1
  Relational Operator : RelationalOperator  Operator=~=  OutDataTypeStr=boolean  RndMeth=Simplest
  Unit Delay : UnitDelay  SampleTime=-1
  Unit Delay1 : UnitDelay  SampleTime=-1
  R2RtSt_Recovery_ini : Outport
  R2RtSt_Recovery_done : Outport  Port=2
  R2Rt_TrgtPoss : Outport  Port=3  VectorParamsAs1DForOutWhenUnconnected=on
  IfVeSMSbSecRwRtStRclCmdSrv_Val_writeRaw : Outport  Port=4
  wires:
  PA_KeSMSwDltTrgtPos_Val8/1 -> R2RtSt_LgrstUpwd_Step3/13
  ModeStCalib_2R/1 -> Bus Selector3/1
  Bus Selector2/6 -> [K_BkReclnUpwdDnwdPosMin]  "<BkReclnUpwdDnwdPosMin>"
  Bus Selector2/2 -> [K_ArmScrnPosMax]  "<ArmScrnPosMax>"
  Bus Selector2/3 -> [K_ArmScrnPosMin]  "<ArmScrnPosMin>"
  Bus Selector2/7 -> [K_FrwdBkwdPos]  "<FrwdBkwdPos>"
  Bus Selector3/1 -> Bus Selector2/1  "<RecoveryMdSecRwRtSt>"
  Bus Selector2/8 -> [K_FrwdBkwdPosMax]  "<FrwdBkwdPosMax>"
  Bus Selector2/5 -> [K_BkReclnUpwdDnwdPosMax]  "<BkReclnUpwdDnwdPosMax>"
  Bus Selector2/9 -> [K_FrwdBkwdPosMin]  "<FrwdBkwdPosMin>"
  Bus Selector2/4 -> [K_BkReclnUpwdDnwdPos]  "<BkReclnUpwdDnwdPos>"
  Bus Selector2/10 -> [K_HdrstUpwdPos]  "<HdrstUpwdPos>"
  Bus Selector2/14 -> [K_LgrstUpwdPosMax]  "<LgrstUpwdPosMax>"
  Bus Selector2/11 -> [K_HdrstUpwdPosMax]  "<HdrstUpwdPosMax>"
  Bus Selector2/13 -> [K_LgrstUpwdPos]  "<LgrstUpwdPos>"
  Bus Selector2/12 -> [K_HdrstUpwdPosMin]  "<HdrstUpwdPosMin>"
  Bus Selector2/17 -> [K_LtwdRtwdPosMax]  "<LtwdRtwdPosMax>"
  Bus Selector2/15 -> [K_LgrstUpwdPosMin]  "<LgrstUpwdPosMin>"
  Bus Selector2/16 -> [K_LtwdRtwdPos]  "<LtwdRtwdPos>"
  Bus Selector2/18 -> [K_LtwdRtwdPosMin]  "<LtwdRtwdPosMin>"
  Bus Selector2/1 -> [K_ArmScrnPos]  "<ArmScrnPos>"
  Bus Selector1/6 -> [R2LtStArmScrnPosV]  "<SecRwRtStArmScrnPosV_Val_read>"
  Bus Selector/6 -> [R2LtStArmScrnPos]  "<SecRwRtStArmScrnPos_Val_read>"
  [KeSMSuMdMotFinshdTm_Val] -> R2RtSt_BkReclnUpwdDnwd_Step1/12
  [KeSMSuMdMotFinshdTm_Val] -> R2RtSt_LgrstUpwd_Step3/12
  PA_KeSMSuModeReqDurgTm_Val/1 -> [Tick]
  PA_KeSMSuMdMotFinshdTm_Val/1 -> [KeSMSuMdMotFinshdTm_Val]
  PA_KeSMSuSecRwStLegrestUpwdDwnwdPosDelta_Val/1 -> [KeSMSuSecRwStLegrestUpwdDwnwdPosDelta_Val]
  PA_KeSMSuSecRwStBackPosDelta_Val/1 -> [KeSMSuSecRwStBackPosDelta_Val]
  PA_KeSMSuSecRwStArmTochPosDelta_Val/1 -> [KeSMSuSecRwStArmTochPosDelta_Val]
  PA_KeSMSuSecRwStLwdRwdPosDelta_Val/1 -> [KeSMSuSecRwStLwdRwdPosDelta_Val]
  PA_KeSMSuSecRwStFwdBkwdPosDelta_Val/1 -> [KeSMSuSecRwStFwdBkwdPosDelta_Val]
  PA_KeSMSwDltTrgtPos_Val1/1 -> Bus Creator/9  "SecRwRtStArmScrnTrgtPos"
  [Step3done_2] -> Logical Operator6/2
  Logical Operator6/1 -> Unit Delay1/1
  [StepEn] -> R2RtSt_BkReclnUpwdDnwd_Step1/2
  [Step3done_1] -> Logical Operator6/1
  [R2Rt_Step3_1_ini] -> Logical Operator1/2
  [R2Rt_Step3_2_ini] -> Logical Operator1/1
  Step1En/1 -> [StepEn]
  PA_KeSMSwDltTrgtPos_Val21/1 -> Bus Creator/4  "SecRwRtStCshnRrUpwdDnwdTrgtPos"
  PA_KeSMSwDltTrgtPos_Val20/1 -> Bus Creator/3  "SecRwRtStCshnFrntUpwdDnwdTrgtPos"
  [R2RtSt_BkReclnUpwdDnwd_TarPos] -> Bus Creator/1  "SecRwRtStBkReclnUpwdDnwdTrgtPos"
  PA_KeSMSwDltTrgtPos_Val19/1 -> Bus Creator/2  "SecRwRtStBlstOtwdInwdTrgtPos"
  [R2RtSt_LgrstUpwd_TarPos] -> Bus Creator/7  "SecRwRtStLgrstUpwdDnwdTrgtPos"
  PA_KeSMSwDltTrgtPos_Val22/1 -> Bus Creator/6  "SecRwRtStHdrstUpwdDnwdTrgtPos"
  PA_KeSMSwDltTrgtPos_Val4/1 -> Bus Creator/8  "SecRwRtStLtwdRtwdTrgtPos"
  PA_KeSMSwDltTrgtPos_Val5/1 -> Bus Creator/5  "SecRwRtStFrwdBkwdTrgtPos"
  Bus Creator/1 -> R2Rt_TrgtPoss/1
  R2RtSt_BkReclnUpwdDnwd_Step1/4 -> Unit Delay/1
  Logical Operator2/1 -> R2RtSt_Recovery_done/1
  Bus Selector/2 -> [SecRwRtStFrwdBkwdPos]  "<IfVeSMSuSecRwRtStFrwdBkwdPos_Val_read>"
  Bus Selector/3 -> [SecRwRtStHPassStUpwdDnwdPos]  "<IfVeSMSuSecRwRtStHPassStUpwdDnwdPos_Val_read>"
  Bus Selector1/5 -> [SecRwRtStLtwdRtwdPosV]  "<IfVeSMSuSecRwRtStLtwdRtwdPosV_Val_read>"
  SecRwRtStPoss/1 -> Bus Selector/1
  Bus Selector/5 -> [SecRwRtStLtwdRtwdPos]  "<IfVeSMSuSecRwRtStLtwdRtwdPos_Val_read>"
  Bus Selector1/4 -> [SecRwRtStLgrstUpwdDnwdPosV]  "<IfVeSMSuSecRwRtStLgrstUpwdDnwdPosV_Val_read>"
  Bus Selector/1 -> [SecRwRtStBkReclnUpwdDnwdPos]  "<IfVeSMSuSecRwRtStBkReclnUpwdDnwdPos_Val_read>"
  Bus Selector1/1 -> [SecRwRtStBkReclnUpwdDnwdPosV]  "<IfVeSMSuSecRwRtStBkReclnUpwdDnwdPosV_Val_read>"
  Bus Selector/4 -> [SecRwRtStLgrstUpwdDnwdPos]  "<IfVeSMSuSecRwRtStLgrstUpwdDnwdPos_Val_read>"
  Bus Selector1/3 -> [SecRwRtStHPassStUpwdDnwdPosV]  "<IfVeSMSuSecRwRtStHPassStUpwdDnwdPosV_Val_read>"
  SecRwRtStPossV/1 -> Bus Selector1/1
  Bus Selector1/2 -> [SecRwRtStFrwdBkwdPosV]  "<IfVeSMSuSecRwRtStFrwdBkwdPosV_Val_read>"
  [K_BkReclnUpwdDnwdPosMax] -> R2RtSt_BkReclnUpwdDnwd_Step1/5
  [Trig] -> R2RtSt_BkReclnUpwdDnwd_Step1/1
  Mode_Trig/1 -> [Trig]
  [KeSMSuSecRwStBackPosDelta_Val] -> R2RtSt_BkReclnUpwdDnwd_Step1/7
  [K_BkReclnUpwdDnwdPosMin] -> R2RtSt_BkReclnUpwdDnwd_Step1/4
  R2RtSt_BkReclnUpwdDnwd_Step1/2 -> [Step1_1_ArrivedTarPos]
  [SecRwRtStBkReclnUpwdDnwdPos] -> R2RtSt_BkReclnUpwdDnwd_Step1/3
  [K_BkReclnUpwdDnwdPos] -> R2RtSt_BkReclnUpwdDnwd_Step1/6
  PA_KeSMSwDltTrgtPos_Val3/1 -> R2RtSt_BkReclnUpwdDnwd_Step1/10
  R2RtSt_BkReclnUpwdDnwd_Step1/3 -> [R2RtSt_BkReclnUpwdDnwd_TarPos]
  [ChildLocker] -> R2RtSt_BkReclnUpwdDnwd_Step1/9
  [Tick] -> R2RtSt_BkReclnUpwdDnwd_Step1/11
  SecRwRtStChldLkRsp_L/1 -> Relational Operator/1
  PA_KeSMSwDltTrgtPos_Val2/1 -> Relational Operator/2
  Relational Operator/1 -> [ChildLocker]
  [Trig] -> R2RtSt_LgrstUpwd_Step3/1
  [K_LgrstUpwdPosMin] -> R2RtSt_LgrstUpwd_Step3/4
  [K_LgrstUpwdPosMax] -> R2RtSt_LgrstUpwd_Step3/5
  [K_LgrstUpwdPos] -> R2RtSt_LgrstUpwd_Step3/6
  [SecRwRtStLgrstUpwdDnwdPos] -> R2RtSt_LgrstUpwd_Step3/3
  [SecRwRtStBkReclnUpwdDnwdPosV] -> R2RtSt_BkReclnUpwdDnwd_Step1/8
  [KeSMSuSecRwStLegrestUpwdDwnwdPosDelta_Val] -> R2RtSt_LgrstUpwd_Step3/7
  [SecRwRtStLgrstUpwdDnwdPosV] -> R2RtSt_LgrstUpwd_Step3/8
  [ChildLocker] -> R2RtSt_LgrstUpwd_Step3/9
  PA_KeSMSwDltTrgtPos_Val12/1 -> R2RtSt_LgrstUpwd_Step3/10
  [Tick] -> R2RtSt_LgrstUpwd_Step3/11
  R2RtSt_LgrstUpwd_Step3/2 -> [Step1_2_ArrivedTarPos]
  R2RtSt_LgrstUpwd_Step3/3 -> [R2RtSt_LgrstUpwd_TarPos]
  R2RtSt_LgrstUpwd_Step3/4 -> [Step3done_2]
  R2RtSt_BkReclnUpwdDnwd_Step1/1 -> [R2Rt_Step3_2_ini]
  Logical Operator1/1 -> R2RtSt_Recovery_ini/1, Logical Operator2/1
  R2RtSt_LgrstUpwd_Step3/1 -> [R2Rt_Step3_1_ini]
  [StepEn] -> R2RtSt_LgrstUpwd_Step3/2
  Unit Delay/1 -> [Step3done_1]
  PA_KeSMSwDltTrgtPos_Val18/1 -> IfVeSMSbSecRwRtStRclCmdSrv_Val_writeRaw/1
  Unit Delay1/1 -> Logical Operator2/2
  StConfig/1 -> Bus Selector4/1
  Bus Selector4/3 -> [FrwdBkwdMovConfig]  "<FrwdBkwdMovConfig>"
  Bus Selector4/5 -> [LtwdRtwdMovConfig]  "<LtwdRtwdMovConfig>"
  Bus Selector4/4 -> [LgrstUpwdMovConfig]  "<LgrstUpwdMovConfig>"
  Bus Selector4/2 -> [ArmTouchMovConfig]  "<ArmTouchMovConfig>"
  Bus Selector4/1 -> [BkReclnUpwdDnwdMovConfig]  "<BkReclnUpwdDnwdMovConfig>"
  [LgrstUpwdMovConfig] -> R2RtSt_LgrstUpwd_Step3/14
  [CntLow] -> R2RtSt_LgrstUpwd_Step3/15
  PA_KeSMSuMdRetryTm1_Val/1 -> [CntLow]
  [BkReclnUpwdDnwdMovConfig] -> R2RtSt_BkReclnUpwdDnwd_Step1/14
  PA_KeSMSwDltTrgtPos_Val6/1 -> R2RtSt_BkReclnUpwdDnwd_Step1/13
  [CntLow] -> R2RtSt_BkReclnUpwdDnwd_Step1/15

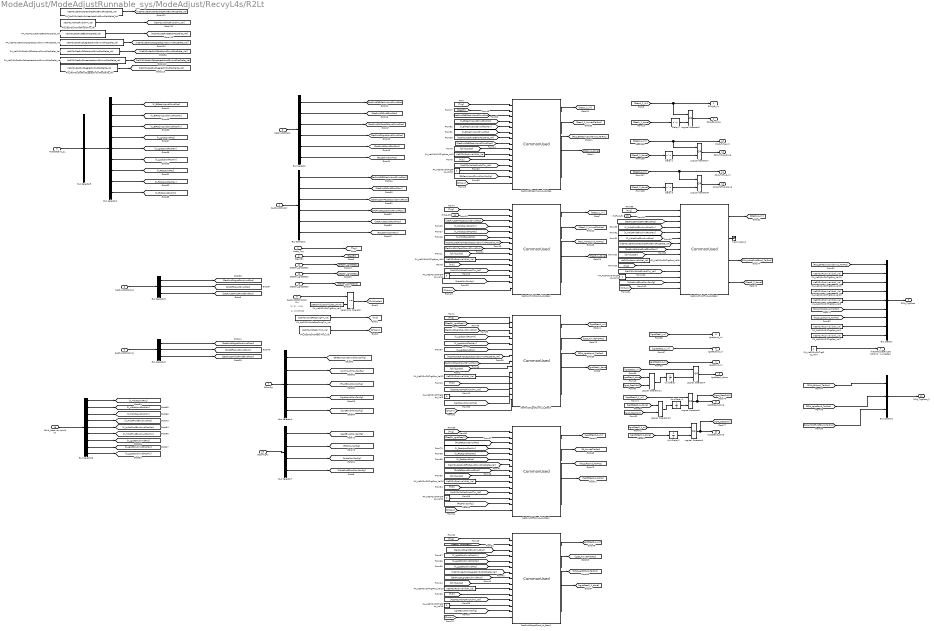
== system ModeAdjust/ModeAdjustRunnable_sys/ModeAdjust/RecvyL4s/R2Lt ==
  note: 2L 扶手屏位置
  note: %1锁，2未锁
  Mode_Trig : Inport
  Step1En : Inport  Port=2
  SecRwLtStsPoss : Inport  Port=3
  SecRwLtStPossV : Inport  Port=4
  SecRwRtStChldLkRsp_L : Inport  Port=5
  ModeStCalib_2L : Inport  Port=6
  StConfig : Inport  Port=7
  SecRwLtStsPoss4s : Inport  Port=8
  SecRwLtStPossV4s : Inport  Port=9
  StConfig4s : Inport  Port=10
  StepEn_LgrstStep1 : Inport  Port=11
  StepEn_LgrstStep2 : Inport  Port=12
  StepEn_LgrstStep3 : Inport  Port=13
  HdUp_En : Inport  Port=14
  HdFwd_En : Inport  Port=15
  Calib_Recovery4sLAdpt : Inport  Port=16
  Bus Creator : BusCreator  Inputs=9  OutDataTypeStr=Bus: SecRwLfSeatPos
  Bus Creator1 : BusCreator  Inputs=3
  Bus Selector : BusSelector  OutputSignals=IfVeSMSuSecRwLtStBkReclnUpwdDnwdPos_Val_read,IfVeSMSuSecRwLtStFrwdBkwdPos_Val_read,IfVeSMSuSecRwLtStHPassStUpwdDnwdPos_Val_read,IfVeSMSuSecRwLtStLgrstUpwdDnwdPos_Val_read,IfVeSMSuSecRwLtStLtwdRtwdPos_Val_read,IfVeSMSuSecRwLtStArmScrnPos_Val_read
  Bus Selector1 : BusSelector  OutputSignals=IfVeSMSuSecRwLtStBkReclnUpwdDnwdPosV_Val_read,IfVeSMSuSecRwLtStFrwdBkwdPosV_Val_read,IfVeSMSuSecRwLtStHPassStUpwdDnwdPosV_Val_read,IfVeSMSuSecRwLtStLgrstUpwdDnwdPosV_Val_read,IfVeSMSuSecRwLtStLtwdRtwdPosV_Val_read,IfVeSMSuSecRwLtStArmScrnPosV_Val_read
  Bus Selector2 : BusSelector  OutputSignals=BkReclnUpwdDnwdPos,BkReclnUpwdDnwdPosMax,BkReclnUpwdDnwdPosMin,LgrstUpwdPos,LgrstUpwdPosMax,LgrstUpwdPosMin,FtrstUpwdDnwdPos,FtrstUpwdDnwdPosMax,FtrstUpwdDnwdPosMin
  Bus Selector3 : BusSelector  OutputSignals=RecvyLSecRwLtSt
  Bus Selector4 : BusSelector  OutputSignals=BkReclnUpwdDnwdMovConfig,ArmTouchMovConfig,FrwdBkwdMovConfig,LgrstUpwdMovConfig,LtwdRtwdMovConfig
  Bus Selector5 : BusSelector  OutputSignals=IfVeSMSuSecRwLtStLgrstOtwdInwdPos_Val_read,IfVeSMSuRrLtStFtUpwdDnwdPos_Val_read,IfVeSMSuSecRwLtStHdrstFrwdBkwdPos_Val_read
  Bus Selector6 : BusSelector  OutputSignals=IfVeSMSuSecRwLtStLgrstOtwdInwdPosV_Val_read,IfVeSMSuRrLtStFtUpwdDnwdPosV_Val_read,IfVeSMSuSecRwLtStHdrstFrwdBkwdPosV_Val_read
  Bus Selector7 : BusSelector  OutputSignals=LgrstExpdMovConfig,FtrstMovConfig,HdrstUpwdDnwdMovConfig,HdrstFrwdBkwdMovConfig
  Bus Selector8 : BusSelector  OutputSignals=HdrstUpwdDnwdPos,HdrstUpwdDnwdPosMax,HdrstUpwdDnwdPosMin,HdrstFrwdBkwdnwdPos,HdrstFrwdBkwdnwdPosMax,HdrstFrwdBkwdnwdPosMin,LgrstOtwdInwdPos,LgrstOtwdInwdPosMax,LgrstOtwdInwdPosMin
  Delay1 : Delay  DelayLength=1
  Delay2 : Delay  DelayLength=1
  Delay3 : Delay  DelayLength=1
  Logical Operator10 : Logic  AllPortsSameDT=off  OutDataTypeStr=boolean
  Logical Operator11 : Logic  AllPortsSameDT=off  OutDataTypeStr=boolean
  Logical Operator{3..8} (6 alike) : Logic  Operator=OR  AllPortsSameDT=off  OutDataTypeStr=boolean
  PA_KeSMSuMdMotFinshdTm_Val : Constant  Value=KeSMSuMdMotFinshdTm_Val
  PA_KeSMSuMdRetryTm1_Val : Constant  Value=KeSMSuMdRetryTm1_Val
  PA_KeSMSuModeReqDurgTm_Val : Constant  Value=KeSMSuModeReqDurgTm_Val
  PA_KeSMSuSecRwStBackPosDelta_Val : Constant  Value=KeSMSuSecRwStBackPosDelta_Val
  PA_KeSMSuSecRwStFtrstUpwdDnwdPosDelta_Val : Constant  Value=KeSMSuSecRwStFtrstUpwdDnwdPosDelta_Val
  PA_KeSMSuSecRwStHeadrestFwdBkwdPosDelta_Val : Constant  Value=KeSMSuSecRwStHeadrestFwdBkwdPosDelta_Val
  PA_KeSMSuSecRwStHeadrestUpwdDwnwdPosDelta_Val : Constant  Value=KeSMSuSecRwStHeadrestUpwdDwnwdPosDelta_Val
  PA_KeSMSuSecRwStLegrestInOutPosDelta_Val : Constant  Value=KeSMSuSecRwStLegrestInOutPosDelta_Val
  PA_KeSMSuSecRwStLegrestUpwdDwnwdPosDelta_Val : Constant  Value=KeSMSuSecRwStLegrestUpwdDwnwdPosDelta_Val
  PA_KeSMSwDltTrgtPos_Val{1,3,5..8,12..13,16,18..20} (12 alike) : Constant  Value=KeSMSwPosInvalidVal_Val
  PA_KeSMSwDltTrgtPos_Val{9..11,15,22,30} (6 alike) : Constant  Value=0  OutDataTypeStr=boolean
  PA_KeSMSwDltTrgtPos_Val2 : Constant  Value=SeatChldLkSt.ChldLkSt_Unlock
  PA_KeSMSwDltTrgtPos_Val4 : Constant  OutDataTypeStr=boolean
  Relational Operator : RelationalOperator  Operator=~=  OutDataTypeStr=boolean  RndMeth=Simplest
  SecRwLtBkRecInUpwd_Lt_Step : Lib/CommonUsed  SystemSampleTime=-1
  SecRwLtHdrstFwd_Lt_Step2 : Lib/CommonUsed  SystemSampleTime=-1
  SecRwLtHdrstUpwd_Lt_Step1 : Lib/CommonUsed  SystemSampleTime=-1
  SecRwLtStFtUpwd_Lt_Step2 : Lib/CommonUsed  SystemSampleTime=-1
  SecRwLtStLgrstOtwd_Lt_Step1 : Lib/CommonUsed  SystemSampleTime=-1
  SecRwLtStLgrstUpwd_Lt_Step3 : Lib/CommonUsed  SystemSampleTime=-1
  Terminator_2 : Terminator
  Unit Delay : UnitDelay  SampleTime=-1
  Unit Delay1 : UnitDelay  SampleTime=-1
  Unit Delay2 : UnitDelay  SampleTime=-1
  R2Lt_Bk_Ini : Outport
  R2Lt_Bk_done : Outport  Port=2
  R2Lt_TrgtPoss : Outport  Port=3  VectorParamsAs1DForOutWhenUnconnected=on
  IfVeSMSuSecRwLtStRclCmdSrv_Val_writeRaw : Outport  Port=4
  lgrstUpwd_ini : Outport  Port=5  VectorParamsAs1DForOutWhenUnconnected=on
  lgrstFtUpwd_ini : Outport  Port=6  VectorParamsAs1DForOutWhenUnconnected=on
  lgrstOtwd_ini : Outport  Port=7  VectorParamsAs1DForOutWhenUnconnected=on
  lgrstStep1_done : Outport  Port=8  VectorParamsAs1DForOutWhenUnconnected=on
  lgrstStep2_done : Outport  Port=9  VectorParamsAs1DForOutWhenUnconnected=on
  lgrstStep3_done : Outport  Port=10  VectorParamsAs1DForOutWhenUnconnected=on
  R2Lt_TrgtPoss_2 : Outport  Port=11  VectorParamsAs1DForOutWhenUnconnected=on
  R2Lt_HdUp_Ini : Outport  Port=12
  R2Lt_HdUp_Done : Outport  Port=13
  R2Lt_HdFwd_Ini : Outport  Port=14
  R2Lt_HdFwd_Done : Outport  Port=15
  wires:
  PA_KeSMSwDltTrgtPos_Val4/1 -> IfVeSMSuSecRwLtStRclCmdSrv_Val_writeRaw/1
  SecRwLtBkRecInUpwd_Lt_Step/4 -> [Step1_1_done]
  SecRwLtStLgrstUpwd_Lt_Step3/1 -> [lgrstStep1_ini]
  [Step1_1_ini] -> Logical Operator3/1, R2Lt_Bk_Ini/1
  [K_BkReclnUpwdDnwdPosMax] -> SecRwLtBkRecInUpwd_Lt_Step/5
  [Trig] -> SecRwLtBkRecInUpwd_Lt_Step/1
  Mode_Trig/1 -> [Trig]
  [KeSMSuSecRwStBackPosDelta_Val] -> SecRwLtBkRecInUpwd_Lt_Step/7
  [K_BkReclnUpwdDnwdPosMin] -> SecRwLtBkRecInUpwd_Lt_Step/4
  SecRwLtBkRecInUpwd_Lt_Step/2 -> [Step1_1_ArrivedTarPos]
  [SecRwLtStBkReclnUpwdDnwdPos] -> SecRwLtBkRecInUpwd_Lt_Step/3
  [K_BkReclnUpwdDnwdPos] -> SecRwLtBkRecInUpwd_Lt_Step/6
  PA_KeSMSwDltTrgtPos_Val3/1 -> SecRwLtBkRecInUpwd_Lt_Step/10
  SecRwLtBkRecInUpwd_Lt_Step/3 -> [R2Lt_BkReclnUpwdDnwd_TarPos]
  [ChildLocker] -> SecRwLtBkRecInUpwd_Lt_Step/9
  [Tick] -> SecRwLtBkRecInUpwd_Lt_Step/11
  Bus Selector1/3 -> [SecRwLtStHPassStUpwdDnwdPosV]  "<IfVeSMSuSecRwLtStHPassStUpwdDnwdPosV_Val_read>"
  Bus Selector/5 -> [SecRwLtStLtwdRtwdPos]  "<IfVeSMSuSecRwLtStLtwdRtwdPos_Val_read>"
  SecRwLtStsPoss/1 -> Bus Selector/1
  Bus Selector1/4 -> [SecRwLtStLgrstUpwdDnwdPosV]  "<IfVeSMSuSecRwLtStLgrstUpwdDnwdPosV_Val_read>"
  SecRwLtStPossV/1 -> Bus Selector1/1
  Bus Selector/3 -> [SecRwLtStHPassStUpwdDnwdPos]  "<IfVeSMSuSecRwLtStHPassStUpwdDnwdPos_Val_read>"
  Bus Selector1/5 -> [SecRwLtStLtwdRtwdPosV]  "<IfVeSMSuSecRwLtStLtwdRtwdPosV_Val_read>"
  Bus Selector/4 -> [SecRwLtStLgrstUpwdDnwdPos]  "<IfVeSMSuSecRwLtStLgrstUpwdDnwdPos_Val_read>"
  Bus Selector/2 -> [SecRwLtStFrwdBkwdPos]  "<IfVeSMSuSecRwLtStFrwdBkwdPos_Val_read>"
  Bus Selector1/1 -> [SecRwLtStBkReclnUpwdDnwdPosV]  "<IfVeSMSuSecRwLtStBkReclnUpwdDnwdPosV_Val_read>"
  Bus Selector1/2 -> [SecRwLtStFrwdBkwdPosV]  "<IfVeSMSuSecRwLtStFrwdBkwdPosV_Val_read>"
  Bus Selector/1 -> [SecRwLtStBkReclnUpwdDnwdPos]  "<IfVeSMSuSecRwLtStBkReclnUpwdDnwdPos_Val_read>"
  SecRwRtStChldLkRsp_L/1 -> Relational Operator/1
  PA_KeSMSwDltTrgtPos_Val2/1 -> Relational Operator/2
  Relational Operator/1 -> [ChildLocker]
  [Trig] -> SecRwLtStLgrstUpwd_Lt_Step3/1
  [StepEn_LgrstStep1] -> SecRwLtStLgrstUpwd_Lt_Step3/2
  [K_LgrstUpwdPosMin] -> SecRwLtStLgrstUpwd_Lt_Step3/4
  [K_LgrstUpwdPosMax] -> SecRwLtStLgrstUpwd_Lt_Step3/5
  [K_LgrstUpwdPos] -> SecRwLtStLgrstUpwd_Lt_Step3/6
  [SecRwLtStLgrstUpwdDnwdPos] -> SecRwLtStLgrstUpwd_Lt_Step3/3
  [SecRwLtStBkReclnUpwdDnwdPosV] -> SecRwLtBkRecInUpwd_Lt_Step/8
  [KeSMSuSecRwStLegrestUpwdDwnwdPosDelta_Val] -> SecRwLtStLgrstUpwd_Lt_Step3/7
  [SecRwLtStLgrstUpwdDnwdPosV] -> SecRwLtStLgrstUpwd_Lt_Step3/8
  [ChildLocker] -> SecRwLtStLgrstUpwd_Lt_Step3/9
  PA_KeSMSwDltTrgtPos_Val12/1 -> SecRwLtStLgrstUpwd_Lt_Step3/10
  [Tick] -> SecRwLtStLgrstUpwd_Lt_Step3/11
  SecRwLtStLgrstUpwd_Lt_Step3/2 -> [lgrst_ArrivedTarPos]
  SecRwLtStLgrstUpwd_Lt_Step3/3 -> [R2Lt_LgrstUpwd_TarPos]
  SecRwLtStLgrstUpwd_Lt_Step3/4 -> [lgrstStep1_done]
  SecRwLtBkRecInUpwd_Lt_Step/1 -> [Step1_1_ini]
  [R2Lt_HdrstUpwd_TarPos] -> Bus Creator/6  "SecRwLtStHdrstUpwdDnwdTrgtPos"
  Bus Creator/1 -> R2Lt_TrgtPoss/1
  [R2Lt_LgrstUpwd_TarPos] -> Bus Creator/7  "SecRwLtStLgrstUpwdDnwdTrgtPos"
  PA_KeSMSwDltTrgtPos_Val19/1 -> Bus Creator/3  "SecRwLtStCshnFrntUpwdDnwdTrgtPos"
  PA_KeSMSwDltTrgtPos_Val1/1 -> Bus Creator/8  "SecRwLtStLtwdRtwdTrgtPos"
  PA_KeSMSwDltTrgtPos_Val18/1 -> Bus Creator/2  "SecRwLtStBlstOtwdInwdTrgtPos"
  [R2Lt_BkReclnUpwdDnwd_TarPos] -> Bus Creator/1  "SecRwLtStBkReclnUpwdDnwdTrgtPos"
  PA_KeSMSwDltTrgtPos_Val8/1 -> Bus Creator/5  "SecRwLtStFrwdBkwdTrgtPos"
  PA_KeSMSwDltTrgtPos_Val20/1 -> Bus Creator/4  "SecRwLtStCshnRrUpwdDnwdTrgtPos"
  Step1En/1 -> [StepEn]
  Logical Operator3/1 -> R2Lt_Bk_done/1
  [StepEn] -> SecRwLtBkRecInUpwd_Lt_Step/2
  [Step1_1_done] -> Delay2/1
  Delay2/1 -> Logical Operator3/2
  PA_KeSMSuModeReqDurgTm_Val/1 -> [Tick]
  PA_KeSMSwDltTrgtPos_Val7/1 -> Bus Creator/9  "SecRwLtStArmScrnTrgtPos"
  PA_KeSMSuSecRwStBackPosDelta_Val/1 -> [KeSMSuSecRwStBackPosDelta_Val]
  PA_KeSMSuSecRwStLegrestUpwdDwnwdPosDelta_Val/1 -> [KeSMSuSecRwStLegrestUpwdDwnwdPosDelta_Val]
  PA_KeSMSuMdMotFinshdTm_Val/1 -> [KeSMSuMdMotFinshdTm_Val]
  [KeSMSuMdMotFinshdTm_Val] -> SecRwLtBkRecInUpwd_Lt_Step/12
  [KeSMSuMdMotFinshdTm_Val] -> SecRwLtStLgrstUpwd_Lt_Step3/12
  Bus Selector/6 -> [R2LtStArmScrnPos]  "<IfVeSMSuSecRwLtStArmScrnPos_Val_read>"
  Bus Selector1/6 -> [R2LtStArmScrnPosV]  "<IfVeSMSuSecRwLtStArmScrnPosV_Val_read>"
  Bus Selector2/6 -> [K_LgrstUpwdPosMin]  "<LgrstUpwdPosMin>"
  Bus Selector2/4 -> [K_LgrstUpwdPos]  "<LgrstUpwdPos>"
  Bus Selector2/5 -> [K_LgrstUpwdPosMax]  "<LgrstUpwdPosMax>"
  Bus Selector2/1 -> [K_BkReclnUpwdDnwdPos]  "<BkReclnUpwdDnwdPos>"
  Bus Selector2/2 -> [K_BkReclnUpwdDnwdPosMax]  "<BkReclnUpwdDnwdPosMax>"
  Bus Selector3/1 -> Bus Selector2/1  "<RecvyLSecRwLtSt>"
  Bus Selector2/3 -> [K_BkReclnUpwdDnwdPosMin]  "<BkReclnUpwdDnwdPosMin>"
  ModeStCalib_2L/1 -> Bus Selector3/1
  StConfig/1 -> Bus Selector4/1
  Bus Selector4/3 -> [FrwdBkwdMovConfig]  "<FrwdBkwdMovConfig>"
  Bus Selector4/5 -> [LtwdRtwdMovConfig]  "<LtwdRtwdMovConfig>"
  Bus Selector4/4 -> [LgrstUpwdMovConfig]  "<LgrstUpwdMovConfig>"
  Bus Selector4/2 -> [ArmTouchMovConfig]  "<ArmTouchMovConfig>"
  Bus Selector4/1 -> [BkReclnUpwdDnwdMovConfig]  "<BkReclnUpwdDnwdMovConfig>"
  PA_KeSMSwDltTrgtPos_Val9/1 -> SecRwLtStLgrstUpwd_Lt_Step3/13
  [LgrstUpwdMovConfig] -> SecRwLtStLgrstUpwd_Lt_Step3/14
  [BkReclnUpwdDnwdMovConfig] -> SecRwLtBkRecInUpwd_Lt_Step/14
  [HdrstMovConfig] -> SecRwLtHdrstUpwd_Lt_Step1/14
  PA_KeSMSwDltTrgtPos_Val11/1 -> SecRwLtHdrstUpwd_Lt_Step1/13
  [KeSMSuMdMotFinshdTm_Val] -> SecRwLtHdrstUpwd_Lt_Step1/12
  SecRwLtHdrstUpwd_Lt_Step1/4 -> [Step3_1_done]
  SecRwLtHdrstUpwd_Lt_Step1/3 -> [R2Lt_HdrstUpwd_TarPos]
  SecRwLtHdrstUpwd_Lt_Step1/2 -> [Step1_2_ArrivedTarPos]
  [Tick] -> SecRwLtHdrstUpwd_Lt_Step1/11
  PA_KeSMSwDltTrgtPos_Val6/1 -> SecRwLtHdrstUpwd_Lt_Step1/10
  [ChildLocker] -> SecRwLtHdrstUpwd_Lt_Step1/9
  [SecRwLtStHPassStUpwdDnwdPosV] -> SecRwLtHdrstUpwd_Lt_Step1/8
  [KeSMSuSecRwStHeadrestUpwdDwnwdPosDelta_Val] -> SecRwLtHdrstUpwd_Lt_Step1/7
  [SecRwLtStHPassStUpwdDnwdPos] -> SecRwLtHdrstUpwd_Lt_Step1/3
  [K_HdrstUpwdPos] -> SecRwLtHdrstUpwd_Lt_Step1/6
  [K_HdrstUpwdPosMax] -> SecRwLtHdrstUpwd_Lt_Step1/5
  [K_HdrstUpwdPosMin] -> SecRwLtHdrstUpwd_Lt_Step1/4
  HdUp_En/1 -> SecRwLtHdrstUpwd_Lt_Step1/2
  [Trig] -> SecRwLtHdrstUpwd_Lt_Step1/1
  SecRwLtHdrstUpwd_Lt_Step1/1 -> [Step3_1_ini]
  Bus Selector2/9 -> [K_FtrstUpwdPosMin]  "<FtrstUpwdDnwdPosMin>"
  Bus Selector2/8 -> [K_FtrstUpwdPosMax]  "<FtrstUpwdDnwdPosMax>"
  Bus Selector2/7 -> [K_FtrstUpwdPos]  "<FtrstUpwdDnwdPos>"
  PA_KeSMSuSecRwStFtrstUpwdDnwdPosDelta_Val/1 -> [KeSMSuSecRwStFtrstUpwdDnwdPosDelta_Val]
  PA_KeSMSuSecRwStHeadrestUpwdDwnwdPosDelta_Val/1 -> [KeSMSuSecRwStHeadrestUpwdDwnwdPosDelta_Val]
  PA_KeSMSuSecRwStLegrestInOutPosDelta_Val/1 -> [KeSMSuSecRwStLegrestInOutPosDelta_Val]
  SecRwLtStsPoss4s/1 -> Bus Selector5/1
  SecRwLtStPossV4s/1 -> Bus Selector6/1
  Bus Selector5/1 -> [SecRwLtStLgrstOtwdInwdPos]  "<IfVeSMSuSecRwLtStLgrstOtwdInwdPos_Val_read>"
  Bus Selector5/2 -> [RrLtStFtUpwdDnwdPos]  "<IfVeSMSuRrLtStFtUpwdDnwdPos_Val_read>"
  Bus Selector6/1 -> [SecRwLtStLgrstOtwdInwdPosV]  "<IfVeSMSuSecRwLtStLgrstOtwdInwdPosV_Val_read>"
  Bus Selector6/2 -> [RrLtStFtUpwdDnwdPosV]  "<IfVeSMSuRrLtStFtUpwdDnwdPosV_Val_read>"
  [LgrstExpdMovConfig] -> SecRwLtStLgrstOtwd_Lt_Step1/14
  PA_KeSMSwDltTrgtPos_Val15/1 -> SecRwLtStLgrstOtwd_Lt_Step1/13
  [KeSMSuMdMotFinshdTm_Val] -> SecRwLtStLgrstOtwd_Lt_Step1/12
  SecRwLtStLgrstOtwd_Lt_Step1/4 -> [LgrstStep3_1_done]
  SecRwLtStLgrstOtwd_Lt_Step1/3 -> [R2Lt_LgrstOtwd_TarPos]
  SecRwLtStLgrstOtwd_Lt_Step1/2 -> [LgOt_ArrivedTarPos]
  [Tick] -> SecRwLtStLgrstOtwd_Lt_Step1/11
  PA_KeSMSwDltTrgtPos_Val13/1 -> SecRwLtStLgrstOtwd_Lt_Step1/10
  [ChildLocker] -> SecRwLtStLgrstOtwd_Lt_Step1/9
  [SecRwLtStLgrstOtwdInwdPosV] -> SecRwLtStLgrstOtwd_Lt_Step1/8
  [KeSMSuSecRwStLegrestInOutPosDelta_Val] -> SecRwLtStLgrstOtwd_Lt_Step1/7
  [SecRwLtStLgrstOtwdInwdPos] -> SecRwLtStLgrstOtwd_Lt_Step1/3
  [K_LgrstOtwdInwdPos] -> SecRwLtStLgrstOtwd_Lt_Step1/6
  [K_LgrstOtwdInwdPosMax] -> SecRwLtStLgrstOtwd_Lt_Step1/5
  [K_LgrstOtwdInwdPosMin] -> SecRwLtStLgrstOtwd_Lt_Step1/4
  [StepEn_LgrstStep3] -> SecRwLtStLgrstOtwd_Lt_Step1/2
  [Trig] -> SecRwLtStLgrstOtwd_Lt_Step1/1
  SecRwLtStLgrstOtwd_Lt_Step1/1 -> [LgrstStep3_1_ini]
  SecRwLtStFtUpwd_Lt_Step2/1 -> [LgrstStep2_1_ini]
  [Trig] -> SecRwLtStFtUpwd_Lt_Step2/1
  [StepEn_LgrstStep2] -> SecRwLtStFtUpwd_Lt_Step2/2
  [K_FtrstUpwdPosMin] -> SecRwLtStFtUpwd_Lt_Step2/4
  [K_FtrstUpwdPosMax] -> SecRwLtStFtUpwd_Lt_Step2/5
  [K_FtrstUpwdPos] -> SecRwLtStFtUpwd_Lt_Step2/6
  [RrLtStFtUpwdDnwdPos] -> SecRwLtStFtUpwd_Lt_Step2/3
  [KeSMSuSecRwStFtrstUpwdDnwdPosDelta_Val] -> SecRwLtStFtUpwd_Lt_Step2/7
  [RrLtStFtUpwdDnwdPosV] -> SecRwLtStFtUpwd_Lt_Step2/8
  [ChildLocker] -> SecRwLtStFtUpwd_Lt_Step2/9
  PA_KeSMSwDltTrgtPos_Val16/1 -> SecRwLtStFtUpwd_Lt_Step2/10
  [Tick] -> SecRwLtStFtUpwd_Lt_Step2/11
  SecRwLtStFtUpwd_Lt_Step2/2 -> [Ft_ArrivedTarPos]
  SecRwLtStFtUpwd_Lt_Step2/3 -> [R2Lt_FtUpwd_TarPos]
  SecRwLtStFtUpwd_Lt_Step2/4 -> [LgrstStep2_1_done]
  [KeSMSuMdMotFinshdTm_Val] -> SecRwLtStFtUpwd_Lt_Step2/12
  PA_KeSMSwDltTrgtPos_Val22/1 -> SecRwLtStFtUpwd_Lt_Step2/13
  [FtrstMovConfig] -> SecRwLtStFtUpwd_Lt_Step2/14
  StConfig4s/1 -> Bus Selector7/1
  Bus Selector7/1 -> [LgrstExpdMovConfig]  "<LgrstExpdMovConfig>"
  Bus Selector7/2 -> [FtrstMovConfig]  "<FtrstMovConfig>"
  Bus Selector7/3 -> [HdrstMovConfig]  "<HdrstUpwdDnwdMovConfig>"
  PA_KeSMSwDltTrgtPos_Val30/1 -> SecRwLtBkRecInUpwd_Lt_Step/13
  [lgrstStep1_ini] -> lgrstUpwd_ini/1
  [LgrstStep2_1_ini] -> lgrstFtUpwd_ini/1
  [LgrstStep3_1_ini] -> lgrstOtwd_ini/1
  StepEn_LgrstStep1/1 -> [StepEn_LgrstStep1]
  StepEn_LgrstStep2/1 -> [StepEn_LgrstStep2]
  StepEn_LgrstStep3/1 -> [StepEn_LgrstStep3]
  Logical Operator4/1 -> lgrstStep1_done/1
  [lgrstStep1_ini] -> Logical Operator4/1
  Unit Delay/1 -> Logical Operator4/2
  Logical Operator5/1 -> [lgrst_Step2chk], lgrstStep2_done/1
  Unit Delay1/1 -> Logical Operator5/2
  Logical Operator6/1 -> [lgrst_Step3chk], lgrstStep3_done/1
  Unit Delay2/1 -> Logical Operator6/2
  [LgrstStep3_1_done] -> Unit Delay2/1
  [LgrstStep2_1_ini] -> Logical Operator5/1
  [LgrstStep3_1_ini] -> Logical Operator6/1
  Bus Creator1/1 -> R2Lt_TrgtPoss_2/1
  [R2Lt_FtUpwd_TarPos] -> Bus Creator1/1  "RrLtStFtUpwdDnwdTrgtPos"
  [R2Lt_LgrstOtwd_TarPos] -> Bus Creator1/2  "SecRwLtStLgrstOtwdInwdTrgtPos"
  [LgrstStep2_1_done] -> Logical Operator10/1
  Logical Operator10/1 -> Unit Delay1/1
  [lgrst_Step3chk] -> Logical Operator10/2
  [lgrstStep1_done] -> Logical Operator11/1
  [lgrst_Step2chk] -> Logical Operator11/2
  Logical Operator11/1 -> Unit Delay/1
  [CntLow] -> SecRwLtBkRecInUpwd_Lt_Step/15
  [CntLow] -> SecRwLtHdrstUpwd_Lt_Step1/15
  [CntLow] -> SecRwLtStFtUpwd_Lt_Step2/15
  [CntLow] -> SecRwLtStLgrstOtwd_Lt_Step1/15
  [CntLow] -> SecRwLtStLgrstUpwd_Lt_Step3/15
  PA_KeSMSuMdRetryTm1_Val/1 -> [CntLow]
  [R2Lt_HdrstFrwdBkwd_TarPos] -> Bus Creator1/3  "SecRwLtStHdrstFrwdBkwdTrgtPos"
  Bus Selector7/4 -> [HdrstFrwdBkwdMovConfig]  "<HdrstFrwdBkwdMovConfig>"
  Bus Selector5/3 -> [SecRwLtStHdrstFrwdBkwdPos]  "<IfVeSMSuSecRwLtStHdrstFrwdBkwdPos_Val_read>"
  Bus Selector6/3 -> [SecRwLtStHdrstFrwdBkwdPosV]  "<IfVeSMSuSecRwLtStHdrstFrwdBkwdPosV_Val_read>"
  PA_KeSMSuSecRwStHeadrestFwdBkwdPosDelta_Val/1 -> [KeSMSuSecRwStHeadrestFwdBkwdPosDelta_Val]
  [CntLow] -> SecRwLtHdrstFwd_Lt_Step2/15
  [K_HdrstFrwdBkwdnwdPosMax] -> SecRwLtHdrstFwd_Lt_Step2/5
  [HdrstFrwdBkwdMovConfig] -> SecRwLtHdrstFwd_Lt_Step2/14
  [SecRwLtStHdrstFrwdBkwdPosV] -> SecRwLtHdrstFwd_Lt_Step2/8
  [KeSMSuSecRwStHeadrestFwdBkwdPosDelta_Val] -> SecRwLtHdrstFwd_Lt_Step2/7
  [SecRwLtStHdrstFrwdBkwdPos] -> SecRwLtHdrstFwd_Lt_Step2/3
  [K_HdrstFrwdBkwdnwdPos] -> SecRwLtHdrstFwd_Lt_Step2/6
  PA_KeSMSwDltTrgtPos_Val5/1 -> SecRwLtHdrstFwd_Lt_Step2/10
  SecRwLtHdrstFwd_Lt_Step2/3 -> [R2Lt_HdrstFrwdBkwd_TarPos]
  [ChildLocker] -> SecRwLtHdrstFwd_Lt_Step2/9
  SecRwLtHdrstFwd_Lt_Step2/1 -> [Step3_2_ini]
  [Tick] -> SecRwLtHdrstFwd_Lt_Step2/11
  SecRwLtHdrstFwd_Lt_Step2/2 -> Terminator_2/1
  [KeSMSuMdMotFinshdTm_Val] -> SecRwLtHdrstFwd_Lt_Step2/12
  HdFwd_En/1 -> SecRwLtHdrstFwd_Lt_Step2/2
  PA_KeSMSwDltTrgtPos_Val10/1 -> SecRwLtHdrstFwd_Lt_Step2/13
  [K_HdrstFrwdBkwdnwdPosMin] -> SecRwLtHdrstFwd_Lt_Step2/4
  [Trig] -> SecRwLtHdrstFwd_Lt_Step2/1
  SecRwLtHdrstFwd_Lt_Step2/4 -> [Step3_2_done]
  Logical Operator7/1 -> R2Lt_HdUp_Done/1
  [Step3_1_ini] -> Logical Operator7/1, R2Lt_HdUp_Ini/1
  Delay1/1 -> Logical Operator7/2
  Logical Operator8/1 -> R2Lt_HdFwd_Done/1
  Delay3/1 -> Logical Operator8/2
  [Step3_1_done] -> Delay1/1
  [Step3_2_done] -> Delay3/1
  [Step3_2_ini] -> Logical Operator8/1, R2Lt_HdFwd_Ini/1
  Calib_Recovery4sLAdpt/1 -> Bus Selector8/1
  Bus Selector8/1 -> [K_HdrstUpwdPos]  "<HdrstUpwdDnwdPos>"
  Bus Selector8/2 -> [K_HdrstUpwdPosMax]  "<HdrstUpwdDnwdPosMax>"
  Bus Selector8/3 -> [K_HdrstUpwdPosMin]  "<HdrstUpwdDnwdPosMin>"
  Bus Selector8/4 -> [K_HdrstFrwdBkwdnwdPos]  "<HdrstFrwdBkwdnwdPos>"
  Bus Selector8/5 -> [K_HdrstFrwdBkwdnwdPosMax]  "<HdrstFrwdBkwdnwdPosMax>"
  Bus Selector8/6 -> [K_HdrstFrwdBkwdnwdPosMin]  "<HdrstFrwdBkwdnwdPosMin>"
  Bus Selector8/7 -> [K_LgrstOtwdInwdPos]  "<LgrstOtwdInwdPos>"
  Bus Selector8/8 -> [K_LgrstOtwdInwdPosMax]  "<LgrstOtwdInwdPosMax>"
  Bus Selector8/9 -> [K_LgrstOtwdInwdPosMin]  "<LgrstOtwdInwdPosMin>"
